simulink model "sync_gen_test"  (Simulink 7.0)
settings: Solver=ode45  StartTime=0.0  StopTime=10000  RelTol=1e-3
undefined symbols (not defined in the file or in its folder): roach_3Ghz_spec_lib, sync_gen
libraries: xbsIndex_r4 x9, casper_library x2, xps_library x1
settings Model: Creator=sgowda  LastModifiedBy=sgowda

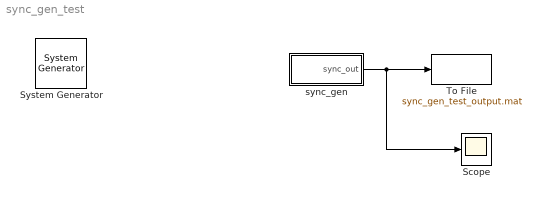
== system sync_gen_test ==
  " System Generator" : xbsIndex_r4/ System Generator  Tag=genX  SystemSampleTime=-1  xilinxfamily=virtex5  part=xc5vlx110t  speed=-1  package=ff1136  synthesis_tool=XST  clock_wrapper=Clock Enables  directory=./roach_spec/sysgen  testbench=off  simulink_period=1  sysclk_period=6.6667  dcm_input_clock_period=100  incr_netlist=off  trim_vbits=Everywhere in SubSystem  dbl_ovrd=According to Block Masks  core_generation=According to Block Masks  run_coregen=off  deprecated_control=off  eval_field=0  block_type=sysgen
      settings: block_version=10.1.1
  Scope : Scope
  To File : ToFile  Filename=sync_gen_test_output.mat  MatrixName=output
  sync_gen : Subsystem  AncestorBlock=roach_3Ghz_spec_lib/sync_gen  mask(sync_gen){sim_acc_len=7, use_soft_reg=off, gen_acc_len=7, fft_size=256, fft_simult_inputs=8, pfb_fir_taps=4, reorder_vec=[5 2 2 2], scale=1}
      mask prompts: sim_acc_len "Simulation Accumulation Length"; use_soft_reg "Set on FPGA using software registers"; gen_acc_len "Synthesized Accumulation Length"; fft_size "FFT Size"; fft_simult_inputs "Simultaneous Inputs (FFT)"; pfb_fir_taps "Taps in pfb_fir (use 1 if no pfb_fir)"; reorder_vec "Reorder Orders (e.g. [2 2 2])"
      mask help:
      | sim_acc_len: The accumulation length (i.e. number of spectra to be summed)  that will be used for simulation. If there is no vector accumulator in your design, use 1.  The simulated accumulation length is used to reduce the amount of time the design takes for simulation.
      |
      | gen_acc_len:  The accumaltion length that will be used for generation.
      |
      | fft_size: The size of the FFT.
      |
      | fft_simult_inputs: The number of data inputs into the FFT
      |
      | pfb_fir_taps: The number of PFB filter taps.  IF no pfb_fir in your design, use 1.
      |
      | reorder_vec: A vector of the orders of the reorder blocks inside the FFT.  In your model, the reorder blocks can be found in fft/fft_biplex/biplex_cplx_unscrambler.  The order should be displayed.
      |
      | scale: The amount to scale the sync period by.
      |
      | SyncPeriod=LCM(reorder_vec)*(acc_num)*(pfb_fir_len)*(fft_size/fft_simult_inputs)
      |
      | Check the box if you would like to use a software register
      | to set the runtime sync period.  NOTE THAT THIS RADIO BUTTON RESETS
      | ITSELF SOMETIMES AFTER IT DRAWS THE SOFTWARE REGISTER, CHECK
      | UNDER THE MASK TO VERIFY.
      mask init:
      | sync_gen_init(gcb, ...
      |     'sim_acc_len', sim_acc_len, ...
      |     'fft_size', fft_size, ...
      |     'gen_acc_len', gen_acc_len, ...
      |     'fft_simult_inputs', fft_simult_inputs,...
      |     'pfb_fir_taps', pfb_fir_taps, ...
      |     'reorder_vec', reorder_vec, ...
      |     'use_soft_reg', use_soft_reg, ...
      |     'scale', scale);
      settings: AttributesFormatString=sim_sync_period=8960
      mask Help:
      | SyncPeriod=LCM(reorder_vec)*(acc_num)*(pfb_fir_len)*(fft_size/fft_simult_inputs)
      | 
      | See CASPER sync pulse memo for more details.
  wires:
  sync_gen/1(sync_out) -> To File/1, Scope/1

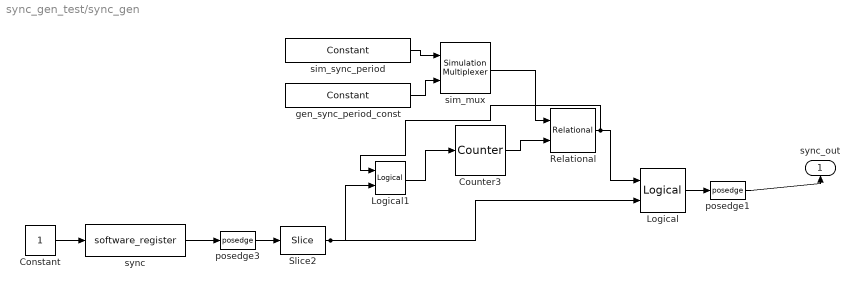
== system sync_gen_test/sync_gen ==
  Constant : Constant  OutDataType=sfix(16)  OutScaling=2^0
  Counter3 : xbsIndex_r4/Counter  cnt_type=Free Running  cnt_to=Inf  operation=Up  start_count=0  cnt_by_val=1  arith_type=Unsigned  n_bits=32  bin_pt=0  load_pin=off  rst=on  en=off  explicit_period=off  period=1  dbl_ovrd=off  use_behavioral_HDL=off  use_rpm=on  block_type=counter
      settings: xl_area=[0, 0, 0, 0, 0, 0, 0]
  Logical : xbsIndex_r4/Logical  logical_function=OR  inputs=2  en=off  latency=0  precision=Full  arith_type=Unsigned  n_bits=8  bin_pt=2  align_bp=on  dbl_ovrd=off  block_type=logical
      settings: xl_area=[0, 0, 0, 0, 0, 0, 0]
  Logical1 : xbsIndex_r4/Logical  logical_function=OR  inputs=2  en=off  latency=0  precision=Full  arith_type=Unsigned  n_bits=8  bin_pt=2  align_bp=on  dbl_ovrd=off  block_type=logical
      settings: xl_area=[0, 0, 0, 0, 0, 0, 0]
  Relational : xbsIndex_r4/Relational  mode=a=b  en=off  latency=1  dbl_ovrd=off  block_type=relational
      settings: xl_area=[0, 0, 0, 0, 0, 0, 0]  block_version=10.1.3
  Slice2 : xbsIndex_r4/Slice  nbits=1  boolean_output=on  mode=Lower Bit Location + Width  bit1=0  base1=MSB of Input  bit0=0  base0=LSB of Input  dbl_ovrd=off  block_type=slice
      settings: infoedit="Extracts a given range of bits from each input sample and presents it at the output.  The output type is ordinarily unsigned with binary point at zero, but can be Boolean when the slice is one bit wide.<P><P>Hardware notes: In hardware this block costs nothing."  block_version=10.1.3
  gen_sync_period_const : xbsIndex_r4/Constant  arith_type=Signed (2's comp)  const=8960  n_bits=32  bin_pt=0  explicit_period=off  period=1  equ=P=C  opselect=C  inp2=PCIN>>17  opr=+  inp1=P  carry=CIN  dbl_ovrd=off  block_type=constant
      settings: block_version=10.1.1
  posedge1 : casper_library/Misc/posedge  Tag=Rising Edge Detector  SystemSampleTime=-1
  posedge3 : casper_library/Misc/posedge  Tag=Rising Edge Detector  SystemSampleTime=-1
  sim_mux : xbsIndex_r4/Simulation Multiplexer  sim_sel=1  hw_sel=2  block_type=simmux
      settings: infoedit="Distinguish input subsystems as \"simulation only\" and \"generation only\".  The input specified For Simulation will be used during Simulink simulation.  The input specified For Generation will be used during code generation.  This block will typically be used on the output of a HW Co-Simulation, Black Box, or ModelSim subsystem.<P><P>Hardware Notes: This block costs nothing."  block_version=10.1.1
  sim_sync_period : xbsIndex_r4/Constant  arith_type=Signed (2's comp)  const=8960  n_bits=32  bin_pt=0  explicit_period=off  period=1  equ=P=C  opselect=C  inp2=PCIN>>17  opr=+  inp1=P  carry=CIN  dbl_ovrd=off  block_type=constant
      settings: block_version=10.1.1
  sync : xps_library/software_register  Tag=xps:sw_reg  SystemSampleTime=-1  io_dir=From Processor  arith_type=Unsigned  bitwidth=32  bin_pt=0  sample_period=1  gw_name=sync_gen_test_sync_gen_sync_user_data_out
      link override sync_gen_test_sync_gen_sync_user_data_out: arith_type=Unsigned  n_bits=32  bin_pt=0  period=1
  sync_out : Outport  Orientation=up  OutDataType=sfix(16)  OutScaling=2^0
  wires:
  gen_sync_period_const/1 -> sim_mux/2
  sim_sync_period/1 -> sim_mux/1
  Constant/1 -> sync/1
  sync/1 -> posedge3/1
  posedge3/1 -> Slice2/1
  Slice2/1 -> Logical1/2, Logical/2
  Logical1/1 -> Counter3/1
  Counter3/1 -> Relational/2
  Relational/1 -> Logical/1, Logical1/1
  Logical/1 -> posedge1/1
  posedge1/1 -> sync_out/1
  sim_mux/1 -> Relational/1
